simulink model "ADCS_Outline"  (R2019a)
settings: Solver=VariableStepAuto  StartTime=0.0  StopTime=duration  MaxStep=step
InitFcn:
  | SC_ODIN_INITIALIZATION
values from neighbouring files (symbols this model uses):
  A = [ v(1) v(4) v(5) v(7);        v(4) v(2) v(6) v(8);        v(5) v(6) v(3) v(9);        v(7) v(8) v(9) v(10) ]    [MagnetometerCalibration.m]    (also in SC_ODIN_INITIALIZATION.m = 0.06; test.m = asin(sin(N)/sin(n)*sin(a)))
  Amag = [0.910186583854  -0.00959593267728  0.00343590491018; -0.00959593267728  1.05471221352  0.0559849466324; 0.00343590491018  0.0559849466324  1.05528532305]    [MagnetometerBias.mat]    (also in MagnetometerCalibration.m = evecs/scale*evecs')
  argentina = [1612.36;-4182.16;-4522.83]    [SC_ODIN_INITIALIZATION.m]
  As = 0.2*0.3    (= 0.06)    [SC_ODIN_INITIALIZATION.m]
  b_mag = block.InputPort(3).Data    [MagnetometerCalibration.m]    (also in SC_ODIN_INITIALIZATION.m = [10;-15.5;-12.2]*1e-6)
  bmag = [1.00003671399e-05 -1.55007781395e-05 -1.22009762149e-05]    [MagnetometerBias.mat]    (also in MagnetometerCalibration.m = centerE)
  breakpoints = data(:,1)    [SC_ODIN_INITIALIZATION.m]
  c = 2.99792458e8    (= 299792458)    [SC_ODIN_INITIALIZATION.m]
  C_I = [0.045 0.0009 -0.00007;        0.0009 0.045 -0.00003;        -0.00007 -0.00003 0.009]    [SC_ODIN_INITIALIZATION.m]
  Cd = 2.0    (= 2)    [SC_ODIN_INITIALIZATION.m]
  controller_sample_rate = 0.5    [SC_ODIN_INITIALIZATION.m]
  D = [ 2 * x,            2 * y,            2 * z,            1 + 0 * x ]    [MagnetometerCalibration.m]    (also in SC_ODIN_INITIALIZATION.m = 0.01*[1;1;1])
  datapx = data(:,2)    [SC_ODIN_INITIALIZATION.m]
  datapy = data(:,3)    [SC_ODIN_INITIALIZATION.m]
  datapz = data(:,4)    [SC_ODIN_INITIALIZATION.m]
  datavx = data(:,5)    [SC_ODIN_INITIALIZATION.m]
  datavy = data(:,6)    [SC_ODIN_INITIALIZATION.m]
  datavz = data(:,7)    [SC_ODIN_INITIALIZATION.m]
  DCM_BT0 = eye(3)    [SC_ODIN_INITIALIZATION.m]
  G = 6.67408e-11    [SC_ODIN_INITIALIZATION.m]
  ground = [1266.06;-4295.81;4526.14]    [SC_ODIN_INITIALIZATION.m]
  I = [Ixx -Ixy -Ixz;      -Ixy Iyy -Iyz;      -Ixz -Iyz Izz]    [SC_ODIN_INITIALIZATION.m]
  invA_mag = block.InputPort(2).Data    [MagnetometerCalibration.m]    (also in SC_ODIN_INITIALIZATION.m = inv(Ellrot/scale*Ellrot'))
  JD_0 = start_day+start_fraction    [SC_ODIN_INITIALIZATION.m]
  Ks = 1367    [SC_ODIN_INITIALIZATION.m]
  L = [0.0000812 -0.0022136 -0.0225868]    [SC_ODIN_INITIALIZATION.m]
  Ls = 0.01*[-3; 3; 5]    [SC_ODIN_INITIALIZATION.m]
  M = 5.9722e24    (= 5.9722e+24)    [SC_ODIN_INITIALIZATION.m]    (also in visualisation.m = uicontrol('Style','text','String',{''},'Position',[710 100+2)
  magnetorquer_tau = 0.02    [SC_ODIN_INITIALIZATION.m]
  magnetorquer_x_saturation = 0.24    [SC_ODIN_INITIALIZATION.m]
  magnetorquer_y_saturation = 0.24    [SC_ODIN_INITIALIZATION.m]
  magnetorquer_z_saturation = 0.13    [SC_ODIN_INITIALIZATION.m]
  namibia = [5659.26;1238.85;-2659.2]    [SC_ODIN_INITIALIZATION.m]
  q = 0.6    [SC_ODIN_INITIALIZATION.m]
  radii = radii .* sgns    [MagnetometerCalibration.m]    (also in SC_ODIN_INITIALIZATION.m = [1;0.9;1.1])
  W0 = [1;0;1-1/240].*pi()/180    [SC_ODIN_INITIALIZATION.m]
  wheel_saturation = 0.23e-3    (= 0.00023)    [SC_ODIN_INITIALIZATION.m]
  wheel_tau = 2    [SC_ODIN_INITIALIZATION.m]
undefined symbols (not defined in the file or in its folder): DiscIntNeverNeededParam, nut80, sun_sensors
libraries: dspmathops x94, vrlib x70, dspsrcs4 x21, realtime_pacer_lib x1, dspsolvers x1, dspinverses x1
(part 6 of 6)

== matlab function ADCS_Outline/Toolbox/EKF Test/MATLAB Function ==
  data: q input; Se input; H output; Be input
function H = H_matrix(q,Se,Be)

%H is the 6x4 matrix jacobian of del h(x) / del x
%It should be a function of q, but in this case, the relation between y
%and x is dependent on the sun and magnetic vectors

H = [ -2*Se(1)*q(4)-2*Se(2)*q(1)+2*Se(3)*q(2)  2*Se(1)*q(1)-2*Se(2)*q(4)+2*Se(3)*q(3) 2*Se(1)*q(2)+2*Se(2)*q(3)+2*Se(3)*q(4) -2*Se(1)*q(3)+2*Se(2)*q(2)+2*Se(3)*q(1);...
       2*Se(1)*q(1)-2*Se(2)*q(4)+2*Se(3)*q(3)  2*Se(1)*q(4)+2*Se(2)*q(1)-2*Se(3)*q(2) 2*Se(1)*q(3)-2*Se(2)*q(2)-2*Se(3)*q(1)  2*Se(1)*q(2)+2*Se(2)*q(3)+2*Se(3)*q(4);...
       2*Se(1)*q(2)+2*Se(2)*q(3)+2*Se(3)*q(4) -2*Se(1)*q(3)+2*Se(2)*q(2)+2*Se(3)*q(1) 2*Se(1)*q(4)+2*Se(2)*q(1)-2*Se(3)*q(2) -2*Se(1)*q(1)+2*Se(2)*q(4)-2*Se(3)*q(3);...
      -2*Be(1)*q(4)-2*Be(2)*q(1)+2*Be(3)*q(2)  2*Be(1)*q(1)-2*Be(2)*q(4)+2*Be(3)*q(3) 2*Be(1)*q(2)+2*Be(2)*q(3)+2*Be(3)*q(4) -2*Be(1)*q(3)+2*Be(2)*q(2)+2*Be(3)*q(1);...
       2*Be(1)*q(1)-2*Be(2)*q(4)+2*Be(3)*q(3)  2*Be(1)*q(4)+2*Be(2)*q(1)-2*Be(3)*q(2) 2*Be(1)*q(3)-2*Be(2)*q(2)-2*Be(3)*q(1)  2*Be(1)*q(2)+2*Be(2)*q(3)+2*Be(3)*q(4);...
       2*Be(1)*q(2)+2*Be(2)*q(3)+2*Be(3)*q(4) -2*Be(1)*q(3)+2*Be(2)*q(2)+2*Be(3)*q(1) 2*Be(1)*q(4)+2*Be(2)*q(1)-2*Be(3)*q(2) -2*Be(1)*q(1)+2*Be(2)*q(4)-2*Be(3)*q(3)];

== matlab function ADCS_Outline/STK Attitude Recording/MATLAB Function ==
  data: u input; y output
function y = fcn(u)

if u==5||u==1
    y=1; %records less data for sun pointing and nadir pointing modes
else
    y=0;
end

== matlab function ADCS_Outline/Toolbox/No Control fast STK attitude recoding/STK Attitude Recording1/DCM to q ==
  data: dcm_inv input; q output
function q = fcn(dcm_inv)

dcm = transpose(dcm_inv);
tr = trace(dcm);

if (tr > 0) 
  S = sqrt(tr+1.0) * 2; % S=4*qw 
  qw = 0.25 * S;
  qx = (dcm(3,2) - dcm(2,3)) / S;
  qy = (dcm(1,3) - dcm(3,1)) / S; 
  qz = (dcm(2,1) - dcm(1,2)) / S; 
elseif ((dcm(1,1) > dcm(2,2)) && (dcm(1,1) > dcm(3,3))) 
  S = sqrt(1.0 + dcm(1,1) - dcm(2,2) - dcm(3,3)) * 2; % S=4*qx 
  qw = (dcm(3,2) - dcm(2,3)) / S;
  qx = 0.25 * S;
  qy = (dcm(1,2) + dcm(2,1)) / S; 
  qz = (dcm(1,3) + dcm(3,1)) / S; 
elseif (dcm(2,2) > dcm(3,3)) 
  S = sqrt(1.0 + dcm(2,2) - dcm(1,1) - dcm(3,3)) * 2; % S=4*qy
  qw = (dcm(1,3) - dcm(3,1)) / S;
  qx = (dcm(1,2) + dcm(2,1)) / S; 
  qy = 0.25 * S;
  qz = (dcm(2,3) + dcm(3,2)) / S; 
 else  
  S = sqrt(1.0 + dcm(3,3) - dcm(1,1) - dcm(2,2)) * 2; % S=4*qz
  qw = (dcm(2,1) - dcm(1,2)) / S;
  qx = (dcm(1,3) + dcm(3,1)) / S;
  qy = (dcm(2,3) + dcm(3,2)) / S;
  qz = 0.25 * S;
end
q = [qx;qy;qz;qw];

== matlab function ADCS_Outline/Toolbox/No Control fast STK attitude recoding/STK Attitude Recording1/MATLAB Function ==
  data: u input; y output
function y = fcn(u)

if u==5||u==1
    y=1;
else
    y=0;
end

== matlab function ADCS_Outline/Toolbox/S//C Kinematics1/Skewed/MATLAB Function ==
  data: u input; y output
function y = fcn(u)
 y = [ 0     u(3) -u(2) u(1); ...
      -u(3)  0     u(1) u(2); ...
       u(2) -u(1)  0    u(3); ...
      -u(1) -u(2) -u(3) 0];

%   y = [0 -u(1)  -u(2)   -u(3); %for (q4 q1 q2 q3) 
%        u(1) 0    u(3)   -u(2) ;
%        u(2) -u(3)  0     u(1);
%        u(3)  u(2) -u(1)  0;];

== matlab function ADCS_Outline/Momentum Control/Momentum Bias/Rotation/MATLAB Function ==
  data: u input; y output
function y = fcn(u)

y = [transpose(u) 0];

== matlab function ADCS_Outline/Toolbox/S//C Kinematics1/  ==
  data: dcm input; q output
function q = fcn(dcm)
tr = trace(dcm);

if (tr > 0) 
  S = sqrt(tr+1.0) * 2; % S=4*qw 
  qw = 0.25 * S;
  qx = (dcm(3,2) - dcm(2,3)) / S;
  qy = (dcm(1,3) - dcm(3,1)) / S; 
  qz = (dcm(2,1) - dcm(1,2)) / S; 
elseif ((dcm(1,1) > dcm(2,2)) && (dcm(1,1) > dcm(3,3))) 
  S = sqrt(1.0 + dcm(1,1) - dcm(2,2) - dcm(3,3)) * 2; % S=4*qx 
  qw = (dcm(3,2) - dcm(2,3)) / S;
  qx = 0.25 * S;
  qy = (dcm(1,2) + dcm(2,1)) / S; 
  qz = (dcm(1,3) + dcm(3,1)) / S; 
elseif (dcm(2,2) > dcm(3,3)) 
  S = sqrt(1.0 + dcm(2,2) - dcm(1,1) - dcm(3,3)) * 2; % S=4*qy
  qw = (dcm(1,3) - dcm(3,1)) / S;
  qx = (dcm(1,2) + dcm(2,1)) / S; 
  qy = 0.25 * S;
  qz = (dcm(2,3) + dcm(3,2)) / S; 
 else  
  S = sqrt(1.0 + dcm(3,3) - dcm(1,1) - dcm(2,2)) * 2; % S=4*qz
  qw = (dcm(2,1) - dcm(1,2)) / S;
  qx = (dcm(1,3) + dcm(3,1)) / S;
  qy = (dcm(2,3) + dcm(3,2)) / S;
  qz = 0.25 * S;
end
q = [qx;qy;qz;qw];

== matlab function ADCS_Outline/Guidance&Determination/Guidance/TRIAD/  ==
  data: dcm input; q output
function q = fcn(dcm)
tr = trace(dcm);

if (tr > 0) 
  S = sqrt(tr+1.0) * 2; % S=4*qw 
  qw = 0.25 * S;
  qx = (dcm(3,2) - dcm(2,3)) / S;
  qy = (dcm(1,3) - dcm(3,1)) / S; 
  qz = (dcm(2,1) - dcm(1,2)) / S; 
elseif ((dcm(1,1) > dcm(2,2)) && (dcm(1,1) > dcm(3,3))) 
  S = sqrt(1.0 + dcm(1,1) - dcm(2,2) - dcm(3,3)) * 2; % S=4*qx 
  qw = (dcm(3,2) - dcm(2,3)) / S;
  qx = 0.25 * S;
  qy = (dcm(1,2) + dcm(2,1)) / S; 
  qz = (dcm(1,3) + dcm(3,1)) / S; 
elseif (dcm(2,2) > dcm(3,3)) 
  S = sqrt(1.0 + dcm(2,2) - dcm(1,1) - dcm(3,3)) * 2; % S=4*qy
  qw = (dcm(1,3) - dcm(3,1)) / S;
  qx = (dcm(1,2) + dcm(2,1)) / S; 
  qy = 0.25 * S;
  qz = (dcm(2,3) + dcm(3,2)) / S; 
 else  
  S = sqrt(1.0 + dcm(3,3) - dcm(1,1) - dcm(2,2)) * 2; % S=4*qz
  qw = (dcm(2,1) - dcm(1,2)) / S;
  qx = (dcm(1,3) + dcm(3,1)) / S;
  qy = (dcm(2,3) + dcm(3,2)) / S;
  qz = 0.25 * S;
end
q = [qx;qy;qz;qw];

== matlab function ADCS_Outline/Toolbox/S//C Kinematics1/MATLAB Function1 ==
  data: u input; y output
function y = fcn(u)

y = [u(4);u(1);u(2);u(3)];

== matlab function ADCS_Outline/Guidance&Determination/Guidance/Guidance ==
  data: Mode input; PointingE output; SE input; PE input; VE input; NE input; AE input; GE input; ConstraintE output; PointingB output; ConstraintB output
function [PointingE, ConstraintE, PointingB, ConstraintB] = Guidance(Mode,SE,PE,VE,NE,AE,GE)

switch Mode
    case 1%Sun  
        PointingE = SE;
        ConstraintE = VE;
        if dot(SE,cross(VE,PE))>0 %if the sun is on the antinormal side
            PointingB = [1;-1;0];%points the sun negative y
        else %if the sun is on the normal side
            PointingB = [-1;-1;0];%points the sun positive y
        end
        ConstraintB = [0;0;1];
    case 2 %Ground
        PointingE = PE;
        ConstraintE = VE;
        PointingB = [0;0;1];
        ConstraintB = [0;1;0];
    case 3 %Imaging Argentina
        PointingE = AE-PE;
        ConstraintE = VE;
        PointingB = [0;1;0];
        ConstraintB = [0;0;1];
    case 4 %Imaging Namibia
        PointingE = VE;
        ConstraintE = NE-PE;
        PointingB = [0;0;1];
        ConstraintB = [0;1;0];    
    otherwise %Nadir
        PointingE = VE;
        ConstraintE = PE;
        PointingB = [0;0;1];
        ConstraintB = [0;-1;0];
  
end

== matlab function ADCS_Outline/Toolbox/MATLAB Function1 ==
  data: CONVERSION input; OUTPUT output; INPUT input; tol input; ichk input
function OUTPUT=SpinCalc(CONVERSION,INPUT,tol,ichk)
%Function for the conversion of one rotation input type to desired output.
%Supported conversion input/output types are as follows:
%   1: Q        Rotation Quaternions
%   2: EV       Euler Vector and rotation angle (degrees)
%   3: DCM      Orthogonal DCM Rotation Matrix
%   4: EA###    Euler angles (12 possible sets) (degrees)
%
%Author: John Fuller
%National Institute of Aerospace
%Hampton, VA 23666
%John.Fuller@nianet.org
%
%Version 1.3
%June 30th, 2009
%
%Version 1.3 updates
%   SpinCalc now detects when input data is too close to Euler singularity, if user is choosing
%   Euler angle output. Prohibits output if middle angle is within 0.1 degree of singularity value.
%~~~~~~~~~~~~~~~~~~~~~~~~~~~~~~~~~~~~~~~~~~~~~~~~~~~~~~~~~~~~~~~~~~~~~~~~~~
%                OUTPUT=SpinCalc(CONVERSION,INPUT,tol,ichk)
%Inputs:
%CONVERSION - Single string value that dictates the type of desired
%             conversion.  The conversion strings are listed below.
%
%   'DCMtoEA###'  'DCMtoEV'    'DCMtoQ'       **for cases that involve   
%   'EA###toDCM'  'EA###toEV'  'EA###toQ'       euler angles, ### should be
%   'EVtoDCM'     'EVtoEA###'  'EVtoQ'          replaced with the proper 
%   'QtoDCM'      'QtoEA###'   'QtoEV'          order desired.  EA321 would
%   'EA###toEA###'                              be Z(yaw)-Y(pitch)-X(roll).
%
%INPUT - matrix or vector that corresponds to the first entry in the
%        CONVERSION string, formatted as follows:
%
%        DCM - 3x3xN multidimensional matrix which pre-multiplies a coordinate
%              frame column vector to calculate its coordinates in the desired 
%              new frame.
%
%        EA### - [psi,theta,phi] (Nx3) row vector list dictating to the first angle
%                rotation (psi), the second (theta), and third (phi) (DEGREES)
%
%        EV - [m1,m2,m3,MU] (Nx4) row vector list dictating the components of euler
%             rotation vector (original coordinate frame) and the Euler 
%             rotation angle about that vector (MU) (DEGREES)
%
%        Q - [q1,q2,q3,q4] (Nx4) row vector list defining quaternion of
%            rotation.  q4 = cos(MU/2) where MU is Euler rotation angle
%
%tol - tolerance value
%ichk - 0 disables warning flags
%          1 enables warning flags (near singularities)
%**NOTE: N corresponds to multiple orientations
%~~~~~~~~~~~~~~~~~~~~~~~~~~~~~~~~~~~~~~~~~~~~~~~~~~~~~~~~~~~~~~~~~~~~~~~~~~
%Output:
%OUTPUT - matrix or vector corresponding to the second entry in the
%         CONVERSION input string, formatted as shown above.
%~~~~~~~~~~~~~~~~~~~~~~~~~~~~~~~~~~~~~~~~~~~~~~~~~~~~~~~~~~~~~~~~~~~~~~~~~~

%Pre-processer to determine type of conversion from CONVERSION string input
%Types are numbered as follows:
%Q=1   EV=2   DCM=3   EA=4
i_type=strfind(lower(CONVERSION),'to');
length=size(CONVERSION,2);
if length>12 || length<4,   %no CONVERSION string can be shorter than 4 or longer than 12 chars
    error('Error: Invalid entry for CONVERSION input string');
end
o_type=length-i_type;
if i_type<5,
    i_type=i_type-1;
else
    i_type=i_type-2;
end
if o_type<5,
    o_type=o_type-1;
else
    o_type=o_type-2;
end
TYPES=cell(1,4);
TYPES{1,1}='Q'; TYPES{1,2}='EV'; TYPES{1,3}='DCM'; TYPES{1,4}='EA';
INPUT_TYPE=TYPES{1,i_type};
OUTPUT_TYPE=TYPES{1,o_type};
clear TYPES
%Confirm input as compared to program interpretation
if i_type~=4 && o_type~=4,  %if input/output are NOT Euler angles
    CC=[INPUT_TYPE,'to',OUTPUT_TYPE];
    if strcmpi(CONVERSION,CC)==0;
        error('Error: Invalid entry for CONVERSION input string');        
    end
else
    if i_type==4,   %if input type is Euler angles, determine the order of rotations
        EULER_order_in=str2double(CONVERSION(1,3:5));
        rot_1_in=floor(EULER_order_in/100);     %first rotation
        rot_2_in=floor((EULER_order_in-rot_1_in*100)/10);   %second rotation
        rot_3_in=(EULER_order_in-rot_1_in*100-rot_2_in*10);   %third rotation
        if rot_1_in<1 || rot_2_in<1 || rot_3_in<1 || rot_1_in>3 || rot_2_in>3 || rot_3_in>3,
            error('Error: Invalid input Euler angle order type (conversion string).');  %check that all orders are between 1 and 3            
        elseif rot_1_in==rot_2_in || rot_2_in==rot_3_in,
            error('Error: Invalid input Euler angle order type (conversion string).');  %check that no 2 consecutive orders are equal (invalid)           
        end
        %check input dimensions to be 1x3x1
        if size(INPUT,2)~=3 || size(INPUT,3)~=1
            error('Error: Input euler angle data vector is not Nx3')            
        end
        %identify singularities        
        input_size = size(INPUT); 
        N = input_size(1); 

        % Identify singularities (second Euler angle out of range) 
        EA2 = INPUT(:,2); % (Nx1) 2nd Euler angle(s) 
        ZEROS = zeros(N,1); % (Nx1) 
        ONES = ones(N,1); % (Nx1) 
        if rot_1_in==rot_3_in % Type 2 rotation (1st and 3rd rotations about same axis) 
            if any(EA2>180*ONES) || any(EA2<ZEROS)
                error('Second input Euler angle(s) outside 0 to 180 degree range') 
            elseif any(EA2>=178*ONES) || any(EA2<=2*ONES)
                if ichk==1 
                    errordlg('Warning: Second input Euler angle(s) near a singularity (0 or 180 degrees).') 
                end 
            end 
        else % Type 1 rotation (rotations about three distinct axes) 
            if any(abs(EA2)>=90*ONES) 
                error('Second input Euler angle(s) outside -90 to 90 degree range') 
            elseif any(abs(EA2)>88*ONES) 
                if ichk==1 
                    errordlg('Warning: Second input Euler angle(s) near a singularity (-90 or 90 degrees).') 
                end 
            end 
        end   
    end
    if o_type==4,   %if output type is Euler angles, determine order of rotations
        EULER_order_out=str2double(CONVERSION(1,length-2:length));
        rot_1_out=floor(EULER_order_out/100);   %first rotation
        rot_2_out=floor((EULER_order_out-rot_1_out*100)/10);    %second rotation
        rot_3_out=(EULER_order_out-rot_1_out*100-rot_2_out*10); %third rotation
        if rot_1_out<1 || rot_2_out<1 || rot_3_out<1 || rot_1_out>3 || rot_2_out>3 || rot_3_out>3,
            error('Error: Invalid output Euler angle order type (conversion string).'); %check that all orders are between 1 and 3           
        elseif rot_1_out==rot_2_out || rot_2_out==rot_3_out,
            error('Error: Invalid output Euler angle order type (conversion string).'); %check that no 2 consecutive orders are equal
        end
    end        
    if i_type==4 && o_type~=4,  %if input are euler angles but not output
        CC=['EA',num2str(EULER_order_in),'to',OUTPUT_TYPE]; %construct program conversion string for checking against user input
    elseif o_type==4 && i_type~=4,  %if output are euler angles but not input
        CC=[INPUT_TYPE,'to','EA',num2str(EULER_order_out)]; %construct program conversion string for checking against user input
    elseif i_type==4 && o_type==4,  %if both input and output are euler angles
        CC=['EA',num2str(EULER_order_in),'to','EA',num2str(EULER_order_out)];   %construct program conversion string
    end
    if strcmpi(CONVERSION,CC)==0; %check program conversion string against user input to confirm the conversion command
        error('Error: Invalid entry for CONVERSION input string');
    end
end
clear i_type o_type CC

%From the input, determine the quaternions that uniquely describe the
%rotation prescribed by that input.  The output will be calculated in the
%second portion of the code from these quaternions.
switch INPUT_TYPE
    case 'DCM'
        if size(INPUT,1)~=3 || size(INPUT,2)~=3  %check DCM dimensions
            error('Error: DCM matrix is not 3x3xN');           
        end
        N=size(INPUT,3);    %number of orientations
        %Check if matrix is indeed orthogonal
        perturbed=NaN(3,3,N);
        DCM_flag=0;
        for ii=1:N,
            perturbed(:,:,ii)=abs(INPUT(:,:,ii)*INPUT(:,:,ii)'-eye(3)); %perturbed array shows difference between DCM*DCM' and I
            if abs(det(INPUT(:,:,ii))-1)>tol, %if determinant is off by one more than tol, user is warned.
                if ichk==1,
                    DCM_flag=1;
                end
            end
            if abs(det(INPUT(:,:,ii))+1)<0.05, %if determinant is near -1, DCM is improper
                error('Error: Input DCM(s) improper');           
            end
            if DCM_flag==1,
                errordlg('Warning: Input DCM matrix determinant(s) off from 1 by more than tolerance.')
            end
        end
        DCM_flag=0;
        if ichk==1,
            for kk=1:N,
                for ii=1:3,
                    for jj=1:3,
                        if perturbed(ii,jj,kk)>tol,   %if any difference is larger than tol, user is warned.
                            DCM_flag=1;
                        end
                    end
                end
            end
            if DCM_flag==1,
                fprintf('Warning: Input DCM(s) matrix not orthogonal to precision tolerance.')
            end
        end       
        clear perturbed DCM_flag   
        Q=NaN(4,N);
        for ii=1:N,
            denom=NaN(4,1);
            denom(1)=0.5*sqrt(1+INPUT(1,1,ii)-INPUT(2,2,ii)-INPUT(3,3,ii));
            denom(2)=0.5*sqrt(1-INPUT(1,1,ii)+INPUT(2,2,ii)-INPUT(3,3,ii));
            denom(3)=0.5*sqrt(1-INPUT(1,1,ii)-INPUT(2,2,ii)+INPUT(3,3,ii));
            denom(4)=0.5*sqrt(1+INPUT(1,1,ii)+INPUT(2,2,ii)+INPUT(3,3,ii));        
            %determine which Q equations maximize denominator
            switch find(denom==max(denom),1,'first')  %determines max value of qtests to put in denominator
                case 1
                    Q(1,ii)=denom(1);
                    Q(2,ii)=(INPUT(1,2,ii)+INPUT(2,1,ii))/(4*Q(1,ii));
                    Q(3,ii)=(INPUT(1,3,ii)+INPUT(3,1,ii))/(4*Q(1,ii));
                    Q(4,ii)=(INPUT(2,3,ii)-INPUT(3,2,ii))/(4*Q(1,ii));
                case 2
                    Q(2,ii)=denom(2);
                    Q(1,ii)=(INPUT(1,2,ii)+INPUT(2,1,ii))/(4*Q(2,ii));
                    Q(3,ii)=(INPUT(2,3,ii)+INPUT(3,2,ii))/(4*Q(2,ii));
                    Q(4,ii)=(INPUT(3,1,ii)-INPUT(1,3,ii))/(4*Q(2,ii));
                case 3
                    Q(3,ii)=denom(3);
                    Q(1,ii)=(INPUT(1,3,ii)+INPUT(3,1,ii))/(4*Q(3,ii));
                    Q(2,ii)=(INPUT(2,3,ii)+INPUT(3,2,ii))/(4*Q(3,ii));
                    Q(4,ii)=(INPUT(1,2,ii)-INPUT(2,1,ii))/(4*Q(3,ii));
                case 4
                    Q(4,ii)=denom(4);
                    Q(1,ii)=(INPUT(2,3,ii)-INPUT(3,2,ii))/(4*Q(4,ii));
                    Q(2,ii)=(INPUT(3,1,ii)-INPUT(1,3,ii))/(4*Q(4,ii));
                    Q(3,ii)=(INPUT(1,2,ii)-INPUT(2,1,ii))/(4*Q(4,ii));
            end
        end
        Q=Q';
        clear denom
    case 'EV'  %Euler Vector Input Type
        if size(INPUT,2)~=4 || size(INPUT,3)~=1   %check dimensions
            error('Error: Input euler vector and rotation data matrix is not Nx4')            
        end
        N=size(INPUT,1);
        MU=INPUT(:,4)*pi/180;  %assign mu name for clarity
        if sqrt(INPUT(:,1).^2+INPUT(:,2).^2+INPUT(:,3).^2)-ones(N,1)>tol*ones(N,1),  %check that input m's constitute unit vector
            error('Input euler vector(s) components do not constitute a unit vector')            
        end
        if MU<zeros(N,1) || MU>2*pi*ones(N,1), %check if rotation about euler vector is between 0 and 360
            error('Input euler rotation angle(s) not between 0 and 360 degrees')
        end
        Q=[INPUT(:,1).*sin(MU/2),INPUT(:,2).*sin(MU/2),INPUT(:,3).*sin(MU/2),cos(MU/2)];   %quaternion
        clear m1 m2 m3 MU
    case 'EA'        
        psi=INPUT(:,1)*pi/180;  theta=INPUT(:,2)*pi/180;  phi=INPUT(:,3)*pi/180;
        N=size(INPUT,1);    %number of orientations
        %Pre-calculate cosines and sines of the half-angles for conversion.
        c1=cos(psi./2); c2=cos(theta./2); c3=cos(phi./2);
        s1=sin(psi./2); s2=sin(theta./2); s3=sin(phi./2);
        c13=cos((psi+phi)./2);  s13=sin((psi+phi)./2);
        c1_3=cos((psi-phi)./2);  s1_3=sin((psi-phi)./2);
        c3_1=cos((phi-psi)./2);  s3_1=sin((phi-psi)./2);
        if EULER_order_in==121,
            Q=[c2.*s13,s2.*c1_3,s2.*s1_3,c2.*c13];
        elseif EULER_order_in==232,
            Q=[s2.*s1_3,c2.*s13,s2.*c1_3,c2.*c13];
        elseif EULER_order_in==313;
            Q=[s2.*c1_3,s2.*s1_3,c2.*s13,c2.*c13];
        elseif EULER_order_in==131,
            Q=[c2.*s13,s2.*s3_1,s2.*c3_1,c2.*c13];
        elseif EULER_order_in==212,
            Q=[s2.*c3_1,c2.*s13,s2.*s3_1,c2.*c13];
        elseif EULER_order_in==323,
            Q=[s2.*s3_1,s2.*c3_1,c2.*s13,c2.*c13];
        elseif EULER_order_in==123,
            Q=[s1.*c2.*c3+c1.*s2.*s3,c1.*s2.*c3-s1.*c2.*s3,c1.*c2.*s3+s1.*s2.*c3,c1.*c2.*c3-s1.*s2.*s3];
        elseif EULER_order_in==231,
            Q=[c1.*c2.*s3+s1.*s2.*c3,s1.*c2.*c3+c1.*s2.*s3,c1.*s2.*c3-s1.*c2.*s3,c1.*c2.*c3-s1.*s2.*s3];
        elseif EULER_order_in==312,
            Q=[c1.*s2.*c3-s1.*c2.*s3,c1.*c2.*s3+s1.*s2.*c3,s1.*c2.*c3+c1.*s2.*s3,c1.*c2.*c3-s1.*s2.*s3];
        elseif EULER_order_in==132,
            Q=[s1.*c2.*c3-c1.*s2.*s3,c1.*c2.*s3-s1.*s2.*c3,c1.*s2.*c3+s1.*c2.*s3,c1.*c2.*c3+s1.*s2.*s3];
        elseif EULER_order_in==213,
            Q=[c1.*s2.*c3+s1.*c2.*s3,s1.*c2.*c3-c1.*s2.*s3,c1.*c2.*s3-s1.*s2.*c3,c1.*c2.*c3+s1.*s2.*s3];
        elseif EULER_order_in==321,
            Q=[c1.*c2.*s3-s1.*s2.*c3,c1.*s2.*c3+s1.*c2.*s3,s1.*c2.*c3-c1.*s2.*s3,c1.*c2.*c3+s1.*s2.*s3];
        else
            error('Error: Invalid input Euler angle order type (conversion string)');            
        end
        clear c1 s1 c2 s2 c3 s3 c13 s13 c1_3 s1_3 c3_1 s3_1 psi theta phi
    case 'Q'
        if size(INPUT,2)~=4 || size(INPUT,3)~=1
            error('Error: Input quaternion matrix is not Nx4');            
        end
        N=size(INPUT,1);    %number of orientations 
        if ichk==1,
            if abs(sqrt(INPUT(:,1).^2+INPUT(:,2).^2+INPUT(:,3).^2+INPUT(:,4).^2)-ones(N,1))>tol*ones(N,1)
                errordlg('Warning: Input quaternion norm(s) deviate(s) from unity by more than tolerance')
            end 
        end
        Q=INPUT;
end
clear INPUT INPUT_TYPE EULER_order_in

%Normalize quaternions in case of deviation from unity.  User has already
%been warned of deviation.
Qnorms=sqrt(sum(Q.*Q,2));
Q=[Q(:,1)./Qnorms,Q(:,2)./Qnorms,Q(:,3)./Qnorms,Q(:,4)./Qnorms];

switch OUTPUT_TYPE
    case 'DCM'
        Q=reshape(Q',1,4,N);
        OUTPUT=[Q(1,1,:).^2-Q(1,2,:).^2-Q(1,3,:).^2+Q(1,4,:).^2,2*(Q(1,1,:).*Q(1,2,:)+Q(1,3,:).*Q(1,4,:)),2*(Q(1,1,:).*Q(1,3,:)-Q(1,2,:).*Q(1,4,:));
                2*(Q(1,1,:).*Q(1,2,:)-Q(1,3,:).*Q(1,4,:)),-Q(1,1,:).^2+Q(1,2,:).^2-Q(1,3,:).^2+Q(1,4,:).^2,2*(Q(1,2,:).*Q(1,3,:)+Q(1,1,:).*Q(1,4,:));
                2*(Q(1,1,:).*Q(1,3,:)+Q(1,2,:).*Q(1,4,:)),2*(Q(1,2,:).*Q(1,3,:)-Q(1,1,:).*Q(1,4,:)),-Q(1,1,:).^2-Q(1,2,:).^2+Q(1,3,:).^2+Q(1,4,:).^2];
    case 'EV'
        MU=2*atan2(sqrt(sum(Q(:,1:3).*Q(:,1:3),2)),Q(:,4));
        if sin(MU/2)~=zeros(N,1),
            OUTPUT=[Q(:,1)./sin(MU/2),Q(:,2)./sin(MU/2),Q(:,3)./sin(MU/2),MU*180/pi];
        else
            OUTPUT=NaN(N,4);
            for ii=1:N,
                if sin(MU(ii,1)/2)~=0,
                    OUTPUT(ii,1:4)=[Q(ii,1)/sin(MU(ii,1)/2),Q(ii,2)/sin(MU(ii,1)/2),Q(ii,3)/sin(MU(ii,1)/2),MU(ii,1)*180/pi];
                else
                    OUTPUT(ii,1:4)=[1,0,0,MU(ii,1)*180/pi];
                end
            end
        end
    case 'Q'
        OUTPUT=Q;
    case 'EA'
        if EULER_order_out==121,
            psi=atan2((Q(:,1).*Q(:,2)+Q(:,3).*Q(:,4)),(Q(:,2).*Q(:,4)-Q(:,1).*Q(:,3)));
            theta=acos(Q(:,4).^2+Q(:,1).^2-Q(:,2).^2-Q(:,3).^2);
            phi=atan2((Q(:,1).*Q(:,2)-Q(:,3).*Q(:,4)),(Q(:,1).*Q(:,3)+Q(:,2).*Q(:,4)));
	  Euler_type=2;
        elseif EULER_order_out==232;
            psi=atan2((Q(:,1).*Q(:,4)+Q(:,2).*Q(:,3)),(Q(:,3).*Q(:,4)-Q(:,1).*Q(:,2)));
            theta=acos(Q(:,4).^2-Q(:,1).^2+Q(:,2).^2-Q(:,3).^2);
            phi=atan2((Q(:,2).*Q(:,3)-Q(:,1).*Q(:,4)),(Q(:,1).*Q(:,2)+Q(:,3).*Q(:,4)));
	  Euler_type=2;
        elseif EULER_order_out==313;
            psi=atan2((Q(:,1).*Q(:,3)+Q(:,2).*Q(:,4)),(Q(:,1).*Q(:,4)-Q(:,2).*Q(:,3)));
            theta=acos(Q(:,4).^2-Q(:,1).^2-Q(:,2).^2+Q(:,3).^2);
            phi=atan2((Q(:,1).*Q(:,3)-Q(:,2).*Q(:,4)),(Q(:,1).*Q(:,4)+Q(:,2).*Q(:,3)));
	  Euler_type=2;
        elseif EULER_order_out==131;
            psi=atan2((Q(:,1).*Q(:,3)-Q(:,2).*Q(:,4)),(Q(:,1).*Q(:,2)+Q(:,3).*Q(:,4)));
            theta=acos(Q(:,4).^2+Q(:,1).^2-Q(:,2).^2-Q(:,3).^2);
            phi=atan2((Q(:,1).*Q(:,3)+Q(:,2).*Q(:,4)),(Q(:,3).*Q(:,4)-Q(:,1).*Q(:,2)));
	  Euler_type=2;
        elseif EULER_order_out==212;
            psi=atan2((Q(:,1).*Q(:,2)-Q(:,3).*Q(:,4)),(Q(:,1).*Q(:,4)+Q(:,2).*Q(:,3)));
            theta=acos(Q(:,4).^2-Q(:,1).^2+Q(:,2).^2-Q(:,3).^2);
            phi=atan2((Q(:,1).*Q(:,2)+Q(:,3).*Q(:,4)),(Q(:,1).*Q(:,4)-Q(:,2).*Q(:,3)));
	  Euler_type=2;
        elseif EULER_order_out==323;
            psi=atan2((Q(:,2).*Q(:,3)-Q(:,1).*Q(:,4)),(Q(:,1).*Q(:,3)+Q(:,2).*Q(:,4)));
            theta=acos(Q(:,4).^2-Q(:,1).^2-Q(:,2).^2+Q(:,3).^2);
            phi=atan2((Q(:,1).*Q(:,4)+Q(:,2).*Q(:,3)),(Q(:,2).*Q(:,4)-Q(:,1).*Q(:,3)));
	  Euler_type=2;
        elseif EULER_order_out==123;
            psi=atan2(2.*(Q(:,1).*Q(:,4)-Q(:,2).*Q(:,3)),(Q(:,4).^2-Q(:,1).^2-Q(:,2).^2+Q(:,3).^2));
            theta=asin(2.*(Q(:,1).*Q(:,3)+Q(:,2).*Q(:,4)));
            phi=atan2(2.*(Q(:,3).*Q(:,4)-Q(:,1).*Q(:,2)),(Q(:,4).^2+Q(:,1).^2-Q(:,2).^2-Q(:,3).^2));
	  Euler_type=1;
        elseif EULER_order_out==231;
            psi=atan2(2.*(Q(:,2).*Q(:,4)-Q(:,1).*Q(:,3)),(Q(:,4).^2+Q(:,1).^2-Q(:,2).^2-Q(:,3).^2));
            theta=asin(2.*(Q(:,1).*Q(:,2)+Q(:,3).*Q(:,4)));
            phi=atan2(2.*(Q(:,1).*Q(:,4)-Q(:,3).*Q(:,2)),(Q(:,4).^2-Q(:,1).^2+Q(:,2).^2-Q(:,3).^2));
	  Euler_type=1;
        elseif EULER_order_out==312;
            psi=atan2(2.*(Q(:,3).*Q(:,4)-Q(:,1).*Q(:,2)),(Q(:,4).^2-Q(:,1).^2+Q(:,2).^2-Q(:,3).^2));
            theta=asin(2.*(Q(:,1).*Q(:,4)+Q(:,2).*Q(:,3)));
            phi=atan2(2.*(Q(:,2).*Q(:,4)-Q(:,3).*Q(:,1)),(Q(:,4).^2-Q(:,1).^2-Q(:,2).^2+Q(:,3).^2));
	  Euler_type=1;
        elseif EULER_order_out==132;
            psi=atan2(2.*(Q(:,1).*Q(:,4)+Q(:,2).*Q(:,3)),(Q(:,4).^2-Q(:,1).^2+Q(:,2).^2-Q(:,3).^2));
            theta=asin(2.*(Q(:,3).*Q(:,4)-Q(:,1).*Q(:,2)));
            phi=atan2(2.*(Q(:,1).*Q(:,3)+Q(:,2).*Q(:,4)),(Q(:,4).^2+Q(:,1).^2-Q(:,2).^2-Q(:,3).^2));
	  Euler_type=1;
        elseif EULER_order_out==213;
            psi=atan2(2.*(Q(:,1).*Q(:,3)+Q(:,2).*Q(:,4)),(Q(:,4).^2-Q(:,1).^2-Q(:,2).^2+Q(:,3).^2));
            theta=asin(2.*(Q(:,1).*Q(:,4)-Q(:,2).*Q(:,3)));
            phi=atan2(2.*(Q(:,1).*Q(:,2)+Q(:,3).*Q(:,4)),(Q(:,4).^2-Q(:,1).^2+Q(:,2).^2-Q(:,3).^2));
	  Euler_type=1;
        elseif EULER_order_out==321;
            psi=atan2(2.*(Q(:,1).*Q(:,2)+Q(:,3).*Q(:,4)),(Q(:,4).^2+Q(:,1).^2-Q(:,2).^2-Q(:,3).^2));
            theta=asin(2.*(Q(:,2).*Q(:,4)-Q(:,1).*Q(:,3)));
            phi=atan2(2.*(Q(:,1).*Q(:,4)+Q(:,3).*Q(:,2)),(Q(:,4).^2-Q(:,1).^2-Q(:,2).^2+Q(:,3).^2));
	  Euler_type=1;
        else
            error('Error: Invalid output Euler angle order type (conversion string).');           
        end
        if(isreal([psi,theta,phi]))==0,
	        error('Error: Unreal Euler output.  Input resides too close to singularity.  Please choose different output type.')
        end
        OUTPUT=mod([psi,theta,phi]*180/pi,360);  %deg
        if Euler_type==1,
	        sing_chk=find(abs(theta)*180/pi>89.9);
	        sing_chk=sort(sing_chk(sing_chk>0));
	        if size(sing_chk,1)>=1,
		        error('Error: Input rotation #%s resides too close to Type 1 Euler singularity.\nType 1 Euler singularity occurs when second angle is -90 or 90 degrees.\nPlease choose different output type.',num2str(sing_chk(1,1)));
	        end
        elseif Euler_type==2,
	        sing_chk=[find(abs(theta*180/pi)<0.1);find(abs(theta*180/pi-180)<0.1);find(abs(theta*180/pi-360))<0.1];
	        sing_chk=sort(sing_chk(sing_chk>0));
	        if size(sing_chk,1)>=1,
		        error('Error: Input rotation #%s resides too close to Type 2 Euler singularity.\nType 2 Euler singularity occurs when second angle is 0 or 180 degrees.\nPlease choose different output type.',num2str(sing_chk(1,1)));
	        end
        end
end

== matlab function ADCS_Outline/Toolbox/Prediction covariance tester1/MATLAB Function ==
  data: qi input; wi input; step input; I input; Lw input; u input; predictionq output; predictionw output
function [predictionq,predictionw] = fcn(qi,wi,step,I,Lw,u)


invI=inv(I);
step=step/100;
for i=1:1:100 

q = qi.*[-1;-1;-1;1] + .5*[0  wi(3) -wi(2) wi(1);
                         -wi(3)  0   wi(1) wi(2);
                          wi(2) -wi(1) 0   wi(3);
                         -wi(1) -wi(2) -wi(3) 0]*(qi.*[-1;-1;-1;1])*step;
                  
w = wi + (invI*(cross(-wi, I*wi+Lw)-u))*step;

qi=q.*[-1;-1;-1;1];
wi=w;
end
predictionq = q.*[-1;-1;-1;1];
predictionw = w;


% x_check = x_check +[.5*[0  wz -wy wx;
%                       -wz  0   wx wy;
%                        wy -wx 0   wz;
%                       -wx -wy -wz 0]*x_check(1:4)*step;
%                       (invI*(cross(-x_check(5:7), I*x_check(5:7)+Lw)-u))*step];%predict state

== matlab function ADCS_Outline/Guidance&Determination/Body-Earth Estimation/  ==
  data: dcm input; q output
function q = fcn(dcm)
tr = trace(dcm);

if (tr > 0) 
  S = sqrt(tr+1.0) * 2; % S=4*qw 
  qw = 0.25 * S;
  qx = (dcm(3,2) - dcm(2,3)) / S;
  qy = (dcm(1,3) - dcm(3,1)) / S; 
  qz = (dcm(2,1) - dcm(1,2)) / S; 
elseif ((dcm(1,1) > dcm(2,2)) && (dcm(1,1) > dcm(3,3))) 
  S = sqrt(1.0 + dcm(1,1) - dcm(2,2) - dcm(3,3)) * 2; % S=4*qx 
  qw = (dcm(3,2) - dcm(2,3)) / S;
  qx = 0.25 * S;
  qy = (dcm(1,2) + dcm(2,1)) / S; 
  qz = (dcm(1,3) + dcm(3,1)) / S; 
elseif (dcm(2,2) > dcm(3,3)) 
  S = sqrt(1.0 + dcm(2,2) - dcm(1,1) - dcm(3,3)) * 2; % S=4*qy
  qw = (dcm(1,3) - dcm(3,1)) / S;
  qx = (dcm(1,2) + dcm(2,1)) / S; 
  qy = 0.25 * S;
  qz = (dcm(2,3) + dcm(3,2)) / S; 
 else  
  S = sqrt(1.0 + dcm(3,3) - dcm(1,1) - dcm(2,2)) * 2; % S=4*qz
  qw = (dcm(2,1) - dcm(1,2)) / S;
  qx = (dcm(1,3) + dcm(3,1)) / S;
  qy = (dcm(2,3) + dcm(3,2)) / S;
  qz = 0.25 * S;
end
q = [qx;qy;qz;qw];

== matlab function ADCS_Outline/Toolbox/     ==
  data: qa input; q output; qb input
function q = Quatmultiply(qa,qb)

q4 = qa(4)*qb(4) - qa(1)*qb(1) - qa(2)*qb(2) - qa(3)*qb(3);
q1 = qa(4)*qb(1) + qa(1)*qb(4) + qa(2)*qb(3) - qa(3)*qb(2);
q2 = qa(4)*qb(2) - qa(1)*qb(3) + qa(2)*qb(4) + qa(3)*qb(1);
q3 = qa(4)*qb(3) + qa(1)*qb(2) - qa(2)*qb(1) + qa(3)*qb(4);

q = [q1 q2 q3 q4];

== matlab function ADCS_Outline/Guidance&Determination/Rotation/     ==
  data: qa input; q output; qb input
function q = Quatmultiply(qa,qb)

q4 = qa(4)*qb(4) - qa(1)*qb(1) - qa(2)*qb(2) - qa(3)*qb(3);
q1 = qa(4)*qb(1) + qa(1)*qb(4) + qa(2)*qb(3) - qa(3)*qb(2);
q2 = qa(4)*qb(2) - qa(1)*qb(3) + qa(2)*qb(4) + qa(3)*qb(1);
q3 = qa(4)*qb(3) + qa(1)*qb(2) - qa(2)*qb(1) + qa(3)*qb(4);

q = [q1 q2 q3 q4];

== matlab function ADCS_Outline/Guidance&Determination/Rotation/    1 ==
  data: qa input; q output; qb input
function q = Quatmultiply(qa,qb)

q4 = qa(4)*qb(4) - qa(1)*qb(1) - qa(2)*qb(2) - qa(3)*qb(3);
q1 = qa(4)*qb(1) + qa(1)*qb(4) + qa(2)*qb(3) - qa(3)*qb(2);
q2 = qa(4)*qb(2) - qa(1)*qb(3) + qa(2)*qb(4) + qa(3)*qb(1);
q3 = qa(4)*qb(3) + qa(1)*qb(2) - qa(2)*qb(1) + qa(3)*qb(4);

q = [q1 q2 q3 q4];

== matlab function ADCS_Outline/Guidance&Determination/Rotation/MATLAB Function ==
  data: u input; y output
function y = fcn(u)

y = [transpose(u) 0];

== matlab function ADCS_Outline/Toolbox/MATLAB Function2 ==
  data: va1 input; DCM_AB output; va2 input; vb1 input; vb2 input
function DCM_AB = triad(va1,va2,vb1,vb2)

% va1=[Ax;Ay;Az];
% va2=[Bx;By;Bz];
% vb1=[refAx;refAy;refAz];
% vb2=[refBx;refBy;refBz];

va1=va1/norm(va1);
va2=va2/norm(va2);
vb1=vb1/norm(vb1);
vb2=vb2/norm(vb2);

crossa=cross(va1,va2)/norm(cross(va1,va2));
crossb=cross(vb1,vb2)/norm(cross(vb1,vb2));

DCM_AB=[va1 cross(crossa,va1)/norm(cross(crossa,va1)) crossa]*...
       [vb1 cross(crossb,vb1)/norm(cross(crossb,vb1)) crossb].';

== matlab function ADCS_Outline/Reaction Wheels Control/MATLAB Function2 ==
  data: Lw input; Ti input; Tw output
function Tw = saturation_rw(Lw,Ti)

sat1 = abs(Lw(1))/1.6e-3;
sat2 = abs(Lw(2))/1.6e-3;
sat3 = abs(Lw(3))/1.6e-3;

if sat1>1 && Ti(1)*Lw(1)>0
    T1 = 0;
else 
    T1 = Ti(1);
end

if sat2>1 && Ti(2)*Lw(2)>0
    T2 = 0;
else 
    T2 = Ti(2);
end

if sat3>1 && Ti(3)*Lw(3)>0
    T3 = 0;
else 
    T3 = Ti(3);
end

Tw = [T1;T2;T3];

== matlab function ADCS_Outline/Toolbox/MATLAB Function3 ==
  data: q input; YPR output
function YPR = fcn(q)

Y = atan2(2*(q(4)*q(3)+q(1)*q(2)),1-2*(q(2)^2+q(3)^2));
P = asin(2*(q(4)*q(2)-q(3)*q(1)));
R = atan2(2*(q(4)*q(1)+q(2)*q(3)),1-2*(q(1)^2+q(2)^2));

YPR=[Y;P;R];

== matlab function ADCS_Outline/Guidance&Determination/Eclipse Prediction/Eclipse Prediction ==
  data: s input; Eclipse output; p input
function Eclipse = fcn(s,p)

if dot(s,p)/(norm(s)*norm(p))<-0.32556815 %angle greater than 109degrees
    Eclipse = 1;
else
    Eclipse = 0 ;
end

== matlab function ADCS_Outline/Guidance&Determination/TargetFrameVelocity/     ==
  data: qa input; q output; qb input
function q = Quatmultiply(qa,qb)

q4 = qa(4)*qb(4) - qa(1)*qb(1) - qa(2)*qb(2) - qa(3)*qb(3);
q1 = qa(4)*qb(1) + qa(1)*qb(4) + qa(2)*qb(3) - qa(3)*qb(2);
q2 = qa(4)*qb(2) - qa(1)*qb(3) + qa(2)*qb(4) + qa(3)*qb(1);
q3 = qa(4)*qb(3) + qa(1)*qb(2) - qa(2)*qb(1) + qa(3)*qb(4);

q = [q1 q2 q3 q4];

== matlab function ADCS_Outline/Toolbox/S//C Kinematics2/  ==
  data: dcm input; q output
function q = fcn(dcm)
tr = trace(dcm);

if (tr > 0) 
  S = sqrt(tr+1.0) * 2; % S=4*qw 
  qw = 0.25 * S;
  qx = (dcm(3,2) - dcm(2,3)) / S;
  qy = (dcm(1,3) - dcm(3,1)) / S; 
  qz = (dcm(2,1) - dcm(1,2)) / S; 
elseif ((dcm(1,1) > dcm(2,2)) && (dcm(1,1) > dcm(3,3))) 
  S = sqrt(1.0 + dcm(1,1) - dcm(2,2) - dcm(3,3)) * 2; % S=4*qx 
  qw = (dcm(3,2) - dcm(2,3)) / S;
  qx = 0.25 * S;
  qy = (dcm(1,2) + dcm(2,1)) / S; 
  qz = (dcm(1,3) + dcm(3,1)) / S; 
elseif (dcm(2,2) > dcm(3,3)) 
  S = sqrt(1.0 + dcm(2,2) - dcm(1,1) - dcm(3,3)) * 2; % S=4*qy
  qw = (dcm(1,3) - dcm(3,1)) / S;
  qx = (dcm(1,2) + dcm(2,1)) / S; 
  qy = 0.25 * S;
  qz = (dcm(2,3) + dcm(3,2)) / S; 
 else  
  S = sqrt(1.0 + dcm(3,3) - dcm(1,1) - dcm(2,2)) * 2; % S=4*qz
  qw = (dcm(2,1) - dcm(1,2)) / S;
  qx = (dcm(1,3) + dcm(3,1)) / S;
  qy = (dcm(2,3) + dcm(3,2)) / S;
  qz = 0.25 * S;
end
q = [qx;qy;qz;qw];

== matlab function ADCS_Outline/Toolbox/MATLAB Function4 ==
  data: DCM input; yaw output; pitch output; roll output
function [yaw, pitch, roll] = DCM2euler(DCM)

yaw = atan2(DCM(3,2),DCM(3,3));
pitch = asin(min(1, max(-1, -DCM(3,1))));
roll = atan2(DCM(2,1),DCM(1,1));

end

== matlab function ADCS_Outline/Toolbox/S//C Kinematics2/MATLAB Function1 ==
  data: u input; y output
function y = fcn(u)

y = [u(4);u(1);u(2);u(3)];

== matlab function ADCS_Outline/Toolbox/S//C Kinematics2/Skewed/MATLAB Function ==
  data: u input; y output
function y = fcn(u)
 y = [ 0     u(3) -u(2) u(1); ...
      -u(3)  0     u(1) u(2); ...
       u(2) -u(1)  0    u(3); ...
      -u(1) -u(2) -u(3) 0];

%   y = [0 -u(1)  -u(2)   -u(3); %for (q4 q1 q2 q3) 
%        u(1) 0    u(3)   -u(2) ;
%        u(2) -u(3)  0     u(1);
%        u(3)  u(2) -u(1)  0;];

== matlab function ADCS_Outline/Reaction Wheels Control/MATLAB Function3 ==
  data: q input; YPR output
function YPR = fcn(q)

Y = atan2(2*(q(4)*q(3)+q(1)*q(2)),1-2*(q(2)^2+q(3)^2));
P = asin(2*(q(4)*q(2)-q(3)*q(1)));
R = atan2(2*(q(4)*q(1)+q(2)*q(3)),1-2*(q(1)^2+q(2)^2));

YPR=[Y;P;R];
